simulink model "SharedBuffer_Ex1"  (R2023a)
settings: Solver=VariableStepAuto  StartTime=0.0  StopTime=2  RelTol=1e-3
undefined symbols (not defined in the file): AIE, i, L, ML, nsvh1369, xcvc2602
libraries: vmcUtilities x1, dspsrcs4 x1, aieBasic x1
settings Model: Creator=sdegala  LastModifiedBy=sdegala

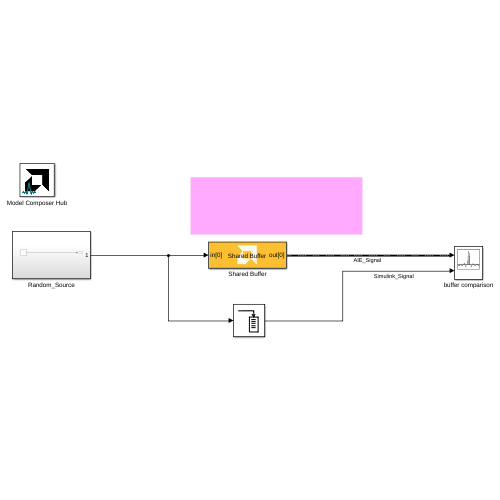
[thumbnail: Simulink's stored preview of the top-level diagram]
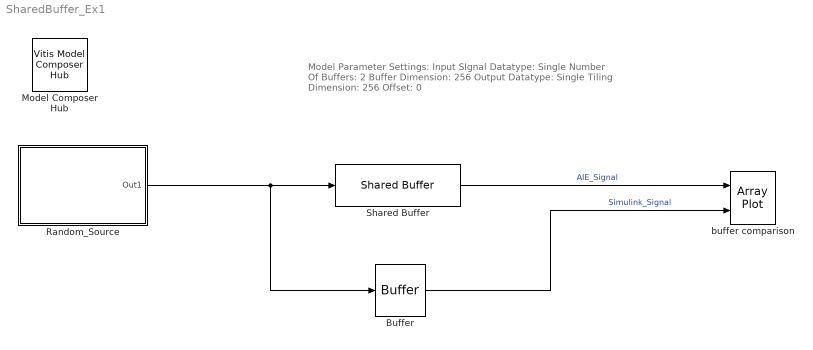
== system SharedBuffer_Ex1 ==
  note: Model Parameter Settings:
      | Input SIgnal Datatype: Single
      | Number Of Buffers: 2
      | Buffer Dimension: 256
      | Output Datatype: Single
      | Tiling Dimension: 256
      | Offset: 0
  Buffer : Buffer  N=256  OutputFrames=off
  Model Composer Hub : vmcUtilities/Vitis Model Composer Hub  Tag=genX  CodeGeneration=off  CompilationType=HDLCompilation  ExportTypeV2=IP Catalog  TargetDirectory=./netlist  exportDesign=off  analyzeDesign=off  validateDesignOnHw=off  ExportType=AI Engines  IpVendor=xilinx.com  IpLibrary=hls  IpVersion=1.0  IpHWLanguage=Verilog  AieCompilerOptions={}  AieSimulatorOptions={}  CreateTestbench=on  TestbenchStackSize=10  RunRtlSim=off  RunCSim=off  RunAieSim=on  AieSimTimeout=50000  RunAieSimProfiling=off  LaunchVitisAnalyzer=off  PlotOutput=off  RunX86Sim=off  X86SimTimeout=10  GenHwImage=off  GenLibadfXo=off  GenHwValidationCode=off  PlatformType=Not Specified  HwSystemType=Baremetal  HwValidationTarget=hw  ProjDevice=xcvc2602-nsvh1369-1LHP-i-L  ProjDevicePart=xcvc2602-nsvh1369-1LHP-i-L  AIEType=AIE-ML  SamplePeriod=-1  ClockFrequency=200  DataPathParallelism=1  xilinxfamily=Kintex7  part=xc7k325t  speed=-3  package=fbg676  directory=./netlist  testbench=off  incr_netlist=off  synthesis_tool=Vivado  clock_wrapper=Clock Enables  dbl_ovrd=According to Block Masks  dcm_input_clock_period=10  sysclk_period=10  simulink_period=1  eval_field=0  LogFileName=/proj/xcoswmktg/robg/git/vmc_examples/gitent/Examples/AIENGINE/DSPlib/Dynamic_FFT/code/model_composer.log  NThreads=4
  Random_Source : Subsystem
  Shared Buffer : aieBasic/Shared Buffer  DataType=float  NumBuffer=2  BufferDim=256  NumInput=1  NumOutput=1  RepetitionCount=0  Input0Tiling=struct('tiling_dimension', 256, 'offset', 0)  Input1Tiling=[]  Input2Tiling=[]  Input3Tiling=[]  Input4Tiling=[]  Input5Tiling=[]  Output0Tiling=struct('tiling_dimension', 256, 'offset', 0)  Output1Tiling=[]  Output2Tiling=[]  Output3Tiling=[]  Output4Tiling=[]  Output5Tiling=[]  InBuffDims={256}  InTilingDims={256}  InOffsets={0}  InTileTraveseDims={}  InTileTraveseStrides={}  InTileTraveseWraps={}  InPacketPortIDs={}  InRepetitions={}  InBoundaryDims={}  OutBuffDims={256}  OutTilingDims={256}  OutOffsets={0}  OutTileTraveseDims={}  OutTileTraveseStrides={}  OutTileTraveseWraps={}  OutPacketPortIDs={}  OutRepetitions={}  OutBoundaryDims={}  BufferDimStr={256}  blockJsonConstraints=[]  deprecateConstraints=0
  buffer comparison : ArrayPlot  NumInputPorts=2  WindowPosition=[4.000000,6.000000,1274.000000,655.000000,]  Visible=on  ScopeFrameLocation=window  PlotType=Line  YLimits=[-0.0933,0.0949]  ShowLegend=on  DefaultConfigurationName=dsp.scopes.ArrayPlotBlockSpecification
  wires:
  Random_Source/1(Out1) -> Buffer/1, Shared Buffer/1
  Buffer/1 -> buffer comparison/2  "Simulink_Signal"
  Shared Buffer/1 -> buffer comparison/1  "AIE_Signal"

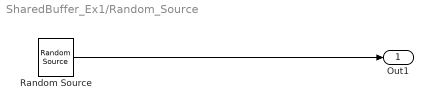
== system SharedBuffer_Ex1/Random_Source ==
  Random Source : dspsrcs4/Random Source  SrcType=Gaussian  NormMethod=Ziggurat  CltLength=12  MinVal=0  MaxVal=1  MeanVal=0  VarVal=0.001  RepMode=Not repeatable  rawSeed=1  IsInherit=off  SampMode=Discrete  SampTime=1/2e6  SampFrame=256  DataType=Single  OutComplex=Real  OutputFrames=off
  Out1 : Outport
  wires:
  Random Source/1 -> Out1/1
